simulink model "T1_INT16_scalar_10_RW_10ms"  (R2021b)
settings: Solver=VariableStepAuto  StartTime=0.0  StopTime=T_sim_end  RelTol=1e-3
values from neighbouring files (symbols this model uses):
  Ts_com = 0.1    [Script_individual_test_init.m]
undefined symbols (not defined in the file or in its folder): PLC_PRG, var01_INT16_scalar_in, var01_INT16_scalar_out, var02_INT16_scalar_in, var02_INT16_scalar_out, var03_INT16_scalar_in, var03_INT16_scalar_out, var04_INT16_scalar_in, var04_INT16_scalar_out, var05_INT16_scalar_in, var05_INT16_scalar_out, var06_INT16_scalar_in, var06_INT16_scalar_out, var07_INT16_scalar_in, var07_INT16_scalar_out, var08_INT16_scalar_in, var08_INT16_scalar_out, var09_INT16_scalar_in, var09_INT16_scalar_out, var10_INT16_scalar_in, var10_INT16_scalar_out
libraries: M1SWBlocks x20
settings Model: Creator=CHSE  LastModifiedBy=CHSE

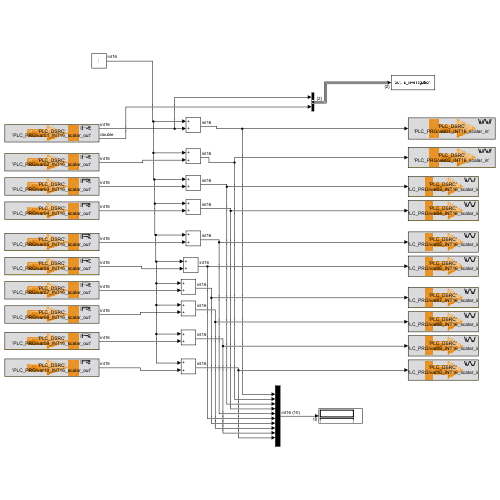
[thumbnail: Simulink's stored preview of the top-level diagram]
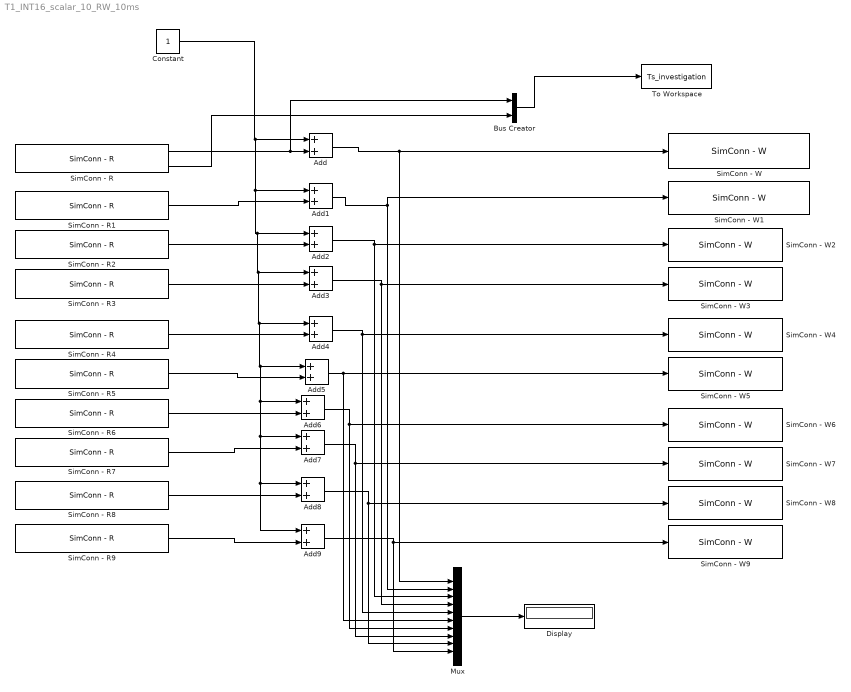
== system T1_INT16_scalar_10_RW_10ms ==
  Add{,1..9} (10 alike) : Sum
  Bus Creator : BusCreator  Inputs=2
  Constant : Constant  OutDataTypeStr=int16  SampleTime=Ts_com
  Display : Display
  Mux : Mux  Inputs=10
  SimConn - R : M1SWBlocks/SimConn Blocks/SimConn - R  connVarName=ConnVar  InswModuleName='PLC_DSRC'  swModuleName=PLC_DSRC  InvarName='PLC_PRG/var01_INT16_scalar_out'  varName=PLC_PRG/var01_INT16_scalar_out  varDataType=int16  enRetOutput=off  enGetTrigger=off  getTrigger=rising  valDurLostConn=Zero  internalVal=0  DataDim=1  enSampTimMon=on  sampleTime=Ts_com
      settings: SourceProductName=Bachmann M1 Software
  SimConn - R1 : M1SWBlocks/SimConn Blocks/SimConn - R  connVarName=ConnVar  InswModuleName='PLC_DSRC'  swModuleName=PLC_DSRC  InvarName='PLC_PRG/var02_INT16_scalar_out'  varName=PLC_PRG/var02_INT16_scalar_out  varDataType=int16  enRetOutput=off  enGetTrigger=off  getTrigger=rising  valDurLostConn=Zero  internalVal=0  DataDim=1  enSampTimMon=off  sampleTime=Ts_com
      settings: SourceProductName=Bachmann M1 Software
  SimConn - R2 : M1SWBlocks/SimConn Blocks/SimConn - R  connVarName=ConnVar  InswModuleName='PLC_DSRC'  swModuleName=PLC_DSRC  InvarName='PLC_PRG/var03_INT16_scalar_out'  varName=PLC_PRG/var03_INT16_scalar_out  varDataType=int16  enRetOutput=off  enGetTrigger=off  getTrigger=rising  valDurLostConn=Zero  internalVal=0  DataDim=1  enSampTimMon=off  sampleTime=Ts_com
      settings: SourceProductName=Bachmann M1 Software
  SimConn - R3 : M1SWBlocks/SimConn Blocks/SimConn - R  connVarName=ConnVar  InswModuleName='PLC_DSRC'  swModuleName=PLC_DSRC  InvarName='PLC_PRG/var04_INT16_scalar_out'  varName=PLC_PRG/var04_INT16_scalar_out  varDataType=int16  enRetOutput=off  enGetTrigger=off  getTrigger=rising  valDurLostConn=Zero  internalVal=0  DataDim=1  enSampTimMon=off  sampleTime=Ts_com
      settings: SourceProductName=Bachmann M1 Software
  SimConn - R4 : M1SWBlocks/SimConn Blocks/SimConn - R  connVarName=ConnVar  InswModuleName='PLC_DSRC'  swModuleName=PLC_DSRC  InvarName='PLC_PRG/var05_INT16_scalar_out'  varName=PLC_PRG/var05_INT16_scalar_out  varDataType=int16  enRetOutput=off  enGetTrigger=off  getTrigger=rising  valDurLostConn=Zero  internalVal=0  DataDim=1  enSampTimMon=off  sampleTime=Ts_com
      settings: SourceProductName=Bachmann M1 Software
  SimConn - R5 : M1SWBlocks/SimConn Blocks/SimConn - R  connVarName=ConnVar  InswModuleName='PLC_DSRC'  swModuleName=PLC_DSRC  InvarName='PLC_PRG/var06_INT16_scalar_out'  varName=PLC_PRG/var06_INT16_scalar_out  varDataType=int16  enRetOutput=off  enGetTrigger=off  getTrigger=rising  valDurLostConn=Zero  internalVal=0  DataDim=1  enSampTimMon=off  sampleTime=Ts_com
      settings: SourceProductName=Bachmann M1 Software
  SimConn - R6 : M1SWBlocks/SimConn Blocks/SimConn - R  connVarName=ConnVar  InswModuleName='PLC_DSRC'  swModuleName=PLC_DSRC  InvarName='PLC_PRG/var07_INT16_scalar_out'  varName=PLC_PRG/var07_INT16_scalar_out  varDataType=int16  enRetOutput=off  enGetTrigger=off  getTrigger=rising  valDurLostConn=Zero  internalVal=0  DataDim=1  enSampTimMon=off  sampleTime=Ts_com
      settings: SourceProductName=Bachmann M1 Software
  SimConn - R7 : M1SWBlocks/SimConn Blocks/SimConn - R  connVarName=ConnVar  InswModuleName='PLC_DSRC'  swModuleName=PLC_DSRC  InvarName='PLC_PRG/var08_INT16_scalar_out'  varName=PLC_PRG/var08_INT16_scalar_out  varDataType=int16  enRetOutput=off  enGetTrigger=off  getTrigger=rising  valDurLostConn=Zero  internalVal=0  DataDim=1  enSampTimMon=off  sampleTime=Ts_com
      settings: SourceProductName=Bachmann M1 Software
  SimConn - R8 : M1SWBlocks/SimConn Blocks/SimConn - R  connVarName=ConnVar  InswModuleName='PLC_DSRC'  swModuleName=PLC_DSRC  InvarName='PLC_PRG/var09_INT16_scalar_out'  varName=PLC_PRG/var09_INT16_scalar_out  varDataType=int16  enRetOutput=off  enGetTrigger=off  getTrigger=rising  valDurLostConn=Zero  internalVal=0  DataDim=1  enSampTimMon=off  sampleTime=Ts_com
      settings: SourceProductName=Bachmann M1 Software
  SimConn - R9 : M1SWBlocks/SimConn Blocks/SimConn - R  connVarName=ConnVar  InswModuleName='PLC_DSRC'  swModuleName=PLC_DSRC  InvarName='PLC_PRG/var10_INT16_scalar_out'  varName=PLC_PRG/var10_INT16_scalar_out  varDataType=int16  enRetOutput=off  enGetTrigger=off  getTrigger=rising  valDurLostConn=Zero  internalVal=0  DataDim=1  enSampTimMon=off  sampleTime=Ts_com
      settings: SourceProductName=Bachmann M1 Software
  SimConn - W : M1SWBlocks/SimConn Blocks/SimConn - W  connVarName=ConnVar  InswModuleName='PLC_DSRC'  swModuleName=PLC_DSRC  InvarName='PLC_PRG/var01_INT16_scalar_in'  varName=PLC_PRG/var01_INT16_scalar_in  varDataType=int16  enRetOutput=off  enGetTrigger=off  getTrigger=rising  enSampTimMon=off
      settings: SourceProductName=Bachmann M1 Software
  SimConn - W1 : M1SWBlocks/SimConn Blocks/SimConn - W  connVarName=ConnVar  InswModuleName='PLC_DSRC'  swModuleName=PLC_DSRC  InvarName='PLC_PRG/var02_INT16_scalar_in'  varName=PLC_PRG/var02_INT16_scalar_in  varDataType=Inherit: auto  enRetOutput=off  enGetTrigger=off  getTrigger=rising  enSampTimMon=off
      settings: SourceProductName=Bachmann M1 Software
  SimConn - W2 : M1SWBlocks/SimConn Blocks/SimConn - W  connVarName=ConnVar  InswModuleName='PLC_DSRC'  swModuleName=PLC_DSRC  InvarName='PLC_PRG/var03_INT16_scalar_in'  varName=PLC_PRG/var03_INT16_scalar_in  varDataType=Inherit: auto  enRetOutput=off  enGetTrigger=off  getTrigger=rising  enSampTimMon=off
      settings: SourceProductName=Bachmann M1 Software
  SimConn - W3 : M1SWBlocks/SimConn Blocks/SimConn - W  connVarName=ConnVar  InswModuleName='PLC_DSRC'  swModuleName=PLC_DSRC  InvarName='PLC_PRG/var04_INT16_scalar_in'  varName=PLC_PRG/var04_INT16_scalar_in  varDataType=Inherit: auto  enRetOutput=off  enGetTrigger=off  getTrigger=rising  enSampTimMon=off
      settings: SourceProductName=Bachmann M1 Software
  SimConn - W4 : M1SWBlocks/SimConn Blocks/SimConn - W  connVarName=ConnVar  InswModuleName='PLC_DSRC'  swModuleName=PLC_DSRC  InvarName='PLC_PRG/var05_INT16_scalar_in'  varName=PLC_PRG/var05_INT16_scalar_in  varDataType=Inherit: auto  enRetOutput=off  enGetTrigger=off  getTrigger=rising  enSampTimMon=off
      settings: SourceProductName=Bachmann M1 Software
  SimConn - W5 : M1SWBlocks/SimConn Blocks/SimConn - W  connVarName=ConnVar  InswModuleName='PLC_DSRC'  swModuleName=PLC_DSRC  InvarName='PLC_PRG/var06_INT16_scalar_in'  varName=PLC_PRG/var06_INT16_scalar_in  varDataType=Inherit: auto  enRetOutput=off  enGetTrigger=off  getTrigger=rising  enSampTimMon=off
      settings: SourceProductName=Bachmann M1 Software
  SimConn - W6 : M1SWBlocks/SimConn Blocks/SimConn - W  connVarName=ConnVar  InswModuleName='PLC_DSRC'  swModuleName=PLC_DSRC  InvarName='PLC_PRG/var07_INT16_scalar_in'  varName=PLC_PRG/var07_INT16_scalar_in  varDataType=Inherit: auto  enRetOutput=off  enGetTrigger=off  getTrigger=rising  enSampTimMon=off
      settings: SourceProductName=Bachmann M1 Software
  SimConn - W7 : M1SWBlocks/SimConn Blocks/SimConn - W  connVarName=ConnVar  InswModuleName='PLC_DSRC'  swModuleName=PLC_DSRC  InvarName='PLC_PRG/var08_INT16_scalar_in'  varName=PLC_PRG/var08_INT16_scalar_in  varDataType=Inherit: auto  enRetOutput=off  enGetTrigger=off  getTrigger=rising  enSampTimMon=off
      settings: SourceProductName=Bachmann M1 Software
  SimConn - W8 : M1SWBlocks/SimConn Blocks/SimConn - W  connVarName=ConnVar  InswModuleName='PLC_DSRC'  swModuleName=PLC_DSRC  InvarName='PLC_PRG/var09_INT16_scalar_in'  varName=PLC_PRG/var09_INT16_scalar_in  varDataType=Inherit: auto  enRetOutput=off  enGetTrigger=off  getTrigger=rising  enSampTimMon=off
      settings: SourceProductName=Bachmann M1 Software
  SimConn - W9 : M1SWBlocks/SimConn Blocks/SimConn - W  connVarName=ConnVar  InswModuleName='PLC_DSRC'  swModuleName=PLC_DSRC  InvarName='PLC_PRG/var10_INT16_scalar_in'  varName=PLC_PRG/var10_INT16_scalar_in  varDataType=Inherit: auto  enRetOutput=off  enGetTrigger=off  getTrigger=rising  enSampTimMon=off
      settings: SourceProductName=Bachmann M1 Software
  To Workspace : ToWorkspace  VariableName=Ts_investigation  SaveFormat=Timeseries  SampleTime=Ts_com
  wires:
  SimConn - R1/1 -> Add1/2
  SimConn - R2/1 -> Add2/2
  SimConn - R3/1 -> Add3/2
  SimConn - R4/1 -> Add4/2
  SimConn - R5/1 -> Add5/2
  SimConn - R6/1 -> Add6/2
  SimConn - R7/1 -> Add7/2
  SimConn - R8/1 -> Add8/2
  SimConn - R9/1 -> Add9/2
  Add1/1 -> Mux/2, SimConn - W1/1
  Add2/1 -> Mux/3, SimConn - W2/1
  Add3/1 -> Mux/4, SimConn - W3/1
  Add4/1 -> Mux/5, SimConn - W4/1
  Add5/1 -> SimConn - W5/1, Mux/6
  Add6/1 -> SimConn - W6/1, Mux/7
  Add7/1 -> SimConn - W7/1, Mux/8
  Add8/1 -> SimConn - W8/1, Mux/9
  Add9/1 -> SimConn - W9/1, Mux/10
  Mux/1 -> Display/1
  Bus Creator/1 -> To Workspace/1
  SimConn - R/2 -> Bus Creator/2
  SimConn - R/1 -> Bus Creator/1, Add/2
  Constant/1 -> Add9/1, Add8/1, Add7/1, Add6/1, Add5/1, Add4/1, Add3/1, Add2/1, Add1/1, Add/1
  Add/1 -> SimConn - W/1, Mux/1
